simulink model "setup"  (R2023b)
settings: Solver=FixedStepAuto  StartTime=0.0  StopTime=10.0  RelTol=1e-3
libraries: arduinolib x7
settings Model: ExtModeTrigDuration=2  Creator=samovar  LastModifiedBy=samovar
settings OptimizationCC: EnhancedBackFolding=on  PassReuseOutputArgsAs=Individual arguments  ZeroExternalMemoryAtStartup=off  ZeroInternalMemoryAtStartup=off  MaxStackSize=64  OptimizeBlockOrder=speed  DifferentSizesBufferReuse=on  OptimizationCustomize=off  EfficientTunableParamExpr=on
settings DebuggingCC: ParameterTunabilityLossMsg=error
settings HardwareCC: ProdBitPerPointer=32  ProdBitPerSizeT=32  ProdBitPerPtrDiffT=32  ProdLargestAtomicInteger=Long  ProdLargestAtomicFloat=Double  ProdWordSize=32  ProdHWDeviceType=ARM Compatible->ARM Cortex  UseEmbeddedCoderFeatures=off  UseSimulinkCoderFeatures=off
settings SFSimCC: MATLABDynamicMemAlloc=off
settings RTWCC: Description=Embedded Coder  SystemTargetFile=ert.tlc  HardwareBoard=ESP32-WROOM(Arduino Compatible)  TLCOptions="-aInlineSetEventsForThisBaseRateFcn=TLC_FALSE -aSuppressMultiTaskScheduler=TLC_FALSE  -aRateBasedStepFcn=0"  TemplateMakefile=ert_default_tmf  Toolchain=ESP32
settings CodeAppCC: ForceParamTrailComments=on  IgnoreCustomStorageClasses=off  OperatorAnnotations=on  SimulinkDataObjDesc=on  SFDataObjDesc=on  InsertBlockDesc=on
settings ERTTargetCC: SupportContinuousTime=on  SupportNonInlinedSFcns=on  SupportVariableSizeSignals=on  ExtModeTransport=3  ExtModeStaticAlloc=on  ExtModeAutomaticAllocSize=off  ExtModeStaticAllocSize=65536  ExtModeMexFile=ext_xcp  ExtModeIntrfLevel=Level2 - Open

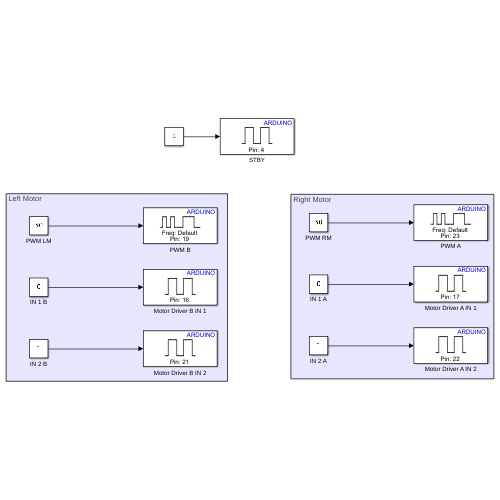
[thumbnail: Simulink's stored preview of the top-level diagram]
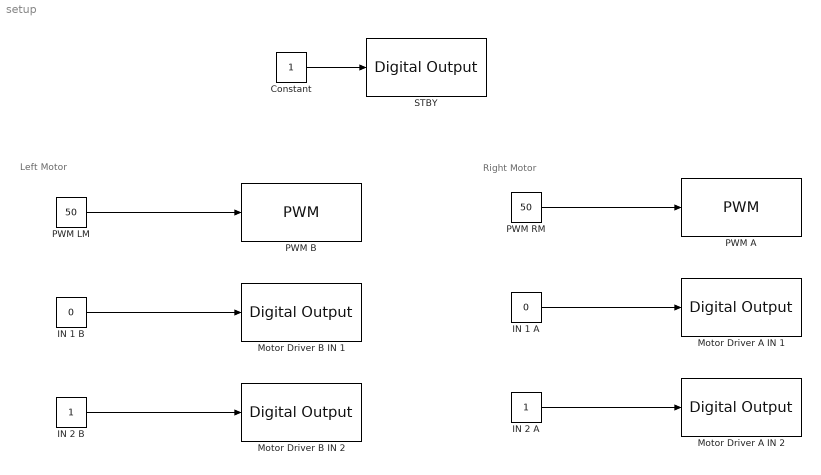
== system setup ==
  note: Left Motor
  note: Right Motor
  Constant : Constant
  IN 1 A : Constant  Value=0
  IN 1 B : Constant  Value=0
  IN 2 A : Constant
  IN 2 B : Constant
  Motor Driver A IN 1 : arduinolib/Digital Output  pinNumber=17  Direction=output  blockPlatform=arduino
  Motor Driver A IN 2 : arduinolib/Digital Output  pinNumber=22  Direction=output  blockPlatform=arduino
  Motor Driver B IN 1 : arduinolib/Digital Output  pinNumber=16  Direction=output  blockPlatform=arduino
  Motor Driver B IN 2 : arduinolib/Digital Output  pinNumber=21  Direction=output  blockPlatform=arduino
  PWM A : arduinolib/PWM  pinNumber=23  frequencyType=Default  desiredFrequency=490.2  achievableFrequency=490.2
  PWM B : arduinolib/PWM  pinNumber=19  frequencyType=Default  desiredFrequency=490.2  achievableFrequency=490.2
  PWM LM : Constant  Value=50
  PWM RM : Constant  Value=50
  STBY : arduinolib/Digital Output  pinNumber=4  Direction=output  blockPlatform=arduino
  wires:
  Constant/1 -> STBY/1
  PWM RM/1 -> PWM A/1
  PWM LM/1 -> PWM B/1
  IN 1 B/1 -> Motor Driver B IN 1/1
  IN 2 B/1 -> Motor Driver B IN 2/1
  IN 2 A/1 -> Motor Driver A IN 2/1
  IN 1 A/1 -> Motor Driver A IN 1/1
